simulink model "v2021_10_27_modello_calcolo_trim_1_semplificato"  (R2020b)
settings: Solver=ode4  StartTime=0.0  StopTime=0.01  FixedStep=0.01  RelTol=1e-3
values from neighbouring files (symbols this model uses):
  alphavec_rad = deg2rad(alphavec)    [v2021_10_27_calcoloAerodinamica.m]
  b = 2.62    [v2021_10_27_calcoloAerodinamica.m]
  betavec_rad = deg2rad(betavec)    [v2021_10_27_calcoloAerodinamica.m]
  c = .32    (= 0.32)    [v2021_10_27_calcoloAerodinamica.m]
  cbar = .32    (= 0.32)    [v2021_10_27_calcoloAerodinamica.m]
  CD0 = 0.024    [v2021_10_27_calcoloAerodinamica.m]
  Clp = -0.5058    [v2021_10_27_calcoloAerodinamica.m]
  CLq = 19.166    [v2021_10_27_calcoloAerodinamica.m]
  Clr = 0.1459    [v2021_10_27_calcoloAerodinamica.m]
  Cmq = -81.796    [v2021_10_27_calcoloAerodinamica.m]
  Cnp = 0.007507    [v2021_10_27_calcoloAerodinamica.m]
  Cnr = -1.2593    [v2021_10_27_calcoloAerodinamica.m]
  CYp = 0.050728    [v2021_10_27_calcoloAerodinamica.m]
  CYr = 0.358925    [v2021_10_27_calcoloAerodinamica.m]
  deltaAtrim = 0    [v2021_10_27_avvioSITL.m]
  deltaEtrim = 0    [v2021_10_27_avvioSITL.m]
  deltaRtrim = 0    [v2021_10_27_avvioSITL.m]
  deltaTtrim = 0.1    [v2021_10_27_avvioSITL.m]
  Dprop = 2*Rprop    (= 0.5334)    [v2021_10_27_calcoloAerodinamica.m]
  Jeng = 0    [v2021_10_27_calcoloAerodinamica.m]
  Jprop = mprop*(Dprop^2)/12    (= 0.00422031414)    [v2021_10_27_calcoloAerodinamica.m]
  matricepolinomi = [0.0816560564319 0.0869820125665 0.0279748858868 -4.51852057237 0.0146653626785 -0.925775006168 8.18052218957e-06 -1.47322908992e-05 7.59644694438e-06 0.00246695371279 9.02269223066e-06 0.000559334242525 ... (126 elements, 6x21)]    [coefficienti_curve_renard.mat]
  q = stato(11)    [measure_F1B.m]
  r = stato(12)    [measure_F1B.m]
  rACtG = rACtP-rGP    [v2021_10_27_calcoloAerodinamica.m]
  rACwG = rACwP-rGP    [v2021_10_27_calcoloAerodinamica.m]
  rAHRSG = rAHRSP-rGP    [v2021_10_27_calcoloAerodinamica.m]
  rho = 1.21330    (= 1.2133)    [v2021_10_27_calcoloAerodinamica.m]
  rLEG = rLEP-rGP    [v2021_10_27_calcoloAerodinamica.m]
  rmglG = rmglP-rGP    [v2021_10_27_calcoloAerodinamica.m]
  rmgrG = rmgrP-rGP    [v2021_10_27_calcoloAerodinamica.m]
  rngG = rngP-rGP    [v2021_10_27_calcoloAerodinamica.m]
  rNPG = rNPP-rGP    [v2021_10_27_calcoloAerodinamica.m]
  rPG = -rGP    [v2021_10_27_calcoloAerodinamica.m]
  Rprop = 0.2667    [v2021_10_27_calcoloAerodinamica.m]
  S = b*cbar    (= 0.8384)    [v2021_10_27_calcoloAerodinamica.m]
  W = m*g    [v2021_10_27_calcoloAerodinamica.m]
  Zeng = rPG(3)    [v2021_10_27_calcoloAerodinamica.m]
undefined symbols (not defined in the file or in its folder): CldA, CLdE, CldR, CmdE, CndA, CndR, CYdA, CYdR, F, J_vec, MIL
libraries: aerolibwind2 x3, shared6dof x1, aerolibasang x1, simulink x1
(part 1 of 2)
settings Model: Creator=Giorgio  LastModifiedBy=39334
settings DataIOCC: ReturnWorkspaceOutputs=off
settings OptimizationCC: BlockReduction=off  OptimizeBlockIOStorage=off  BufferReuse=off  GlobalBufferReuse=off  ExpressionFolding=off  LocalBlockOutputs=off  OptimizeDataStoreBuffers=off  BusAssignmentInplaceUpdate=off
settings DebuggingCC: InitInArrayFormatMsg=none  ArithmeticOperatorsInVariantConditions=warning
settings SFSimCC: CustomCodeUndefinedFunction=UseInterfaceOnly

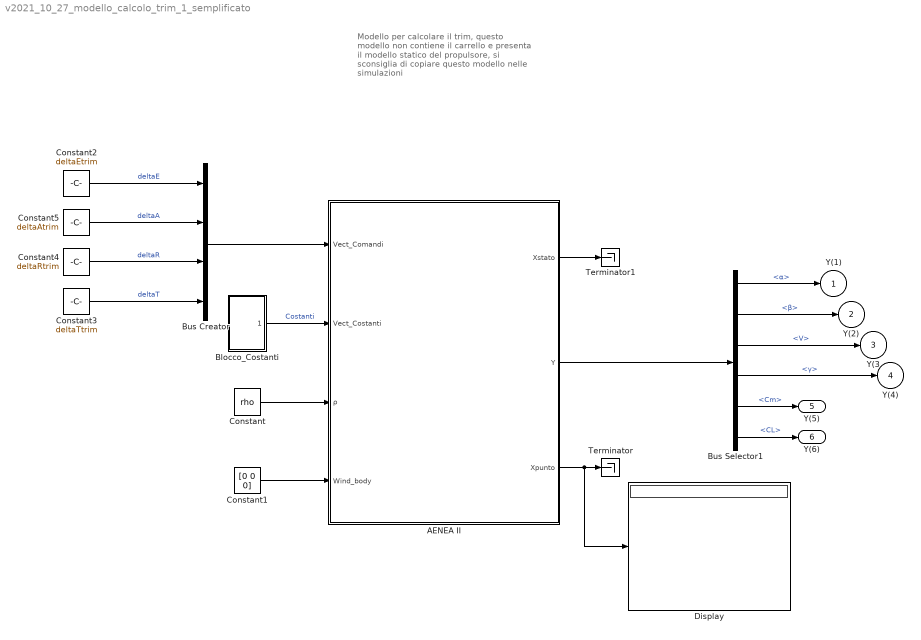
== system v2021_10_27_modello_calcolo_trim_1_semplificato ==
  note: Modello per calcolare il trim, questo modello non contiene il carrello e presenta il modello statico del propulsore, si sconsiglia di copiare questo modello nelle simulazioni
  "AENEA II " : Subsystem
  Blocco_Costanti : Subsystem
  Bus Creator : BusCreator  Inputs=4
  Bus Selector1 : BusSelector  OutputSignals=Vbpolare.α,Vbpolare.β,Vbpolare.V,γ,Cm,CL
  Constant : Constant  Value=rho
  Constant1 : Constant  Value=[0 0 0]
  Constant2 : Constant  Value=deltaEtrim
  Constant3 : Constant  Value=deltaTtrim
  Constant4 : Constant  Value=deltaRtrim
  Constant5 : Constant  Value=deltaAtrim
  Display : Display
  Terminator : Terminator
  Terminator1 : Terminator
  Y(1) : Outport  VectorParamsAs1DForOutWhenUnconnected=off
  Y(2) : Outport  Port=2  VectorParamsAs1DForOutWhenUnconnected=off
  Y(3 : Outport  Port=3  VectorParamsAs1DForOutWhenUnconnected=off
  Y(4) : Outport  Port=4  VectorParamsAs1DForOutWhenUnconnected=off
  Y(5) : Outport  Port=5  VectorParamsAs1DForOutWhenUnconnected=off
  Y(6) : Outport  Port=6  VectorParamsAs1DForOutWhenUnconnected=off
  wires:
  Blocco_Costanti/1(Vect_Costanti) -> "AENEA II "/2(Vect_Costanti)  "Costanti"
  Constant/1 -> "AENEA II "/3(ρ)
  Bus Creator/1 -> "AENEA II "/1(Vect_Comandi)
  Constant5/1 -> Bus Creator/2  "deltaA"
  Constant4/1 -> Bus Creator/3  "deltaR"
  Constant3/1 -> Bus Creator/4  "deltaT"
  Constant2/1 -> Bus Creator/1  "deltaE"
  "AENEA II "/2(Y) -> Bus Selector1/1
  Bus Selector1/1 -> Y(1)/1  "<α>"
  Bus Selector1/2 -> Y(2)/1  "<β>"
  Bus Selector1/3 -> Y(3/1  "<V>"
  Bus Selector1/4 -> Y(4)/1  "<γ>"
  "AENEA II "/1(Xstato) -> Terminator1/1
  Constant1/1 -> "AENEA II "/4(Wind_body)
  "AENEA II "/3(Xpunto) -> Display/1, Terminator/1
  Bus Selector1/5 -> Y(5)/1  "<Cm>"
  Bus Selector1/6 -> Y(6)/1  "<CL>"

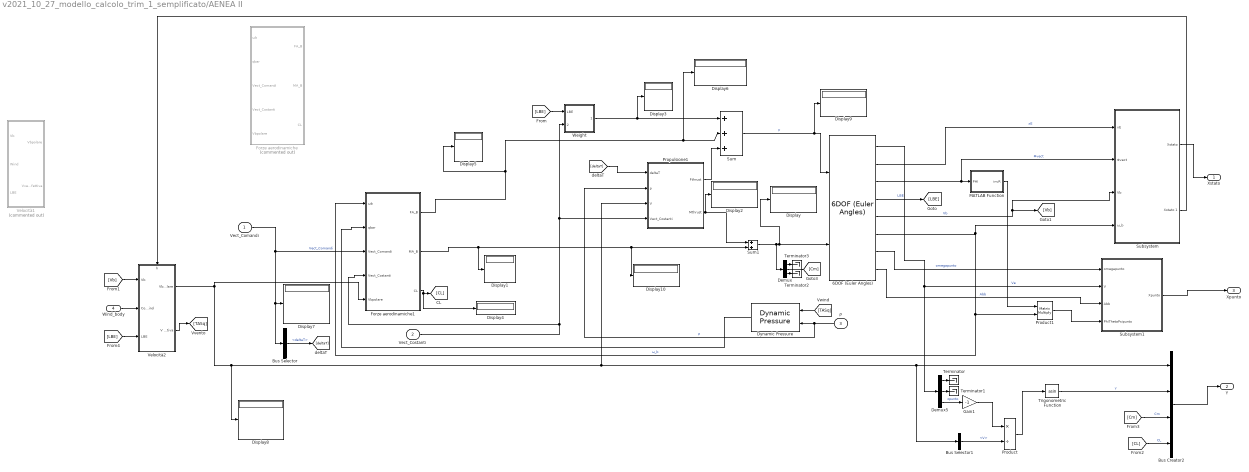
== system v2021_10_27_modello_calcolo_trim_1_semplificato/AENEA II  ==
  Vect_Comandi : Inport
  Vect_Costanti : Inport  Port=2
  ρ : Inport  Port=3
  Wind_body : Inport  Port=4
  6DOF (Euler Angles) : shared6dof/6DOF (Euler Angles)  units=Metric (MKS)  mtype=Fixed  rep=Euler Angles  xme_0=State0.Pos0  Vm_0=State0.Vb0  eul_0=State0.PHI0  pm_0=State0.Omega0  mass_0=m  mass_e=0.5  mass_f=2.0  inertia=I  inertia_e=eye(3)  inertia_f=2*eye(3)  k_quat=1.0  vre_flag=on  abi_flag=off  aMode=aMode  xme_statename=''  Vm_statename=''  eul_statename=''  quat_statename=''  pm_statename=''  mass_statename=''
      settings: SourceProductBaseCode=AE,PW,MT,UV,VE,VP
  Bus Creator2 : BusCreator  Inputs=4
  Bus Selector : BusSelector  OutputSignals=deltaT
  Bus Selector1 : BusSelector  OutputSignals=V
  Demux : Demux  Outputs=3
  Demux5 : Demux  Outputs=3
  Display{,1..10} (11 alike) : Display
  Dynamic Pressure : aerolibasang/Dynamic Pressure
  Forze aerodinamiche : Subsystem  Commented=on
  Forze aerodinamiche1 : Subsystem
  Gain1 : Gain  Gain=-1
  MATLAB Function : MATLAB Function  TreatAsAtomicUnit=on
  Product : Product  Inputs=*/
  Product1 : Product  Multiplication=Matrix(*)
  Propulsione1 : Subsystem
  Subsystem : Subsystem
  Subsystem1 : Subsystem
  Sum : Sum  Inputs=+++
  Sum1 : Sum  Inputs=2
  Terminator{,1..3} (4 alike) : Terminator
  Trigonometric Function : Trigonometry  Operator=asin
  Velocità1 : Subsystem  Commented=on
  Velocità2 : Subsystem
      settings: PortSchema="{\"entries\":[{\"content\":{\"sides\":[{\"content\":{\"connectorIds\":[\"In1\",\"In2\",\"In3\"]},\"type\":\"ConnectorPlacement.EquallySpacedRectSide\",\"uuid\":\"0746aba7-5653-4c82-81e3-16f181e227c2\"},{\"content\":{\"connectorIds\":[\"Out1\",\"Out2\"],\"side\":\"RIGHT\"},\"type\":\"ConnectorPlacement.EquallySpacedRectSide\",\"uuid\":\"8b0f41a9-047a-45e0-b4b5-945564827102\"},{\"content\":{\"connectorIds\":[\"In4\"],\"side\":\"TOP\"},\"type\":\"ConnectorPlacement.EquallySpacedRectSide\",\"uuid\":\"9604396d-4b59-4e8f-8d6f-73032a1dccac\"},{\"content\":{\"connectorIds\":[],\"side\":\"HIDDEN\"},\"type\":\"ConnectorPlacement.EquallySpacedRectSide\",\"uuid\":\"dd1fbc60-e45e-4bfb-a7ae-11fe3343e682\"}]},\"type\":\"ConnectorPlacement.EquallySpacedConnector\",\"uuid\":\"54d3b117-caea-4758-beb0-4ac3e6481041\"}],\"packageUris\":[\"http://schema.mathworks.com/mf0/Connector/R2020b\"],\"version\":\"1.0\"}"
  Weight : Subsystem
  Xstato : Outport  VectorParamsAs1DForOutWhenUnconnected=off
  Y : Outport  Port=2  VectorParamsAs1DForOutWhenUnconnected=off
  Xpunto : Outport  Port=3  VectorParamsAs1DForOutWhenUnconnected=off
  wires:
  Sum/1 -> Display9/1, 6DOF (Euler Angles)/1  "F"
  6DOF (Euler Angles)/5 -> Subsystem/3(Vb), [Vb]  "Vb"
  6DOF (Euler Angles)/6 -> Forze aerodinamiche1/1(ωb), Product1/2, Subsystem/4(ω_b)  "ω_b"
  6DOF (Euler Angles)/4 -> [LBE]  "LBE"
  Forze aerodinamiche1/1(FA_B) -> Sum/2, Display6/1, Display5/1
  Forze aerodinamiche1/2(MA_B) -> Display10/1, Sum1/2, Display1/1
  6DOF (Euler Angles)/1 -> Demux5/1, Subsystem1/2(V)  "Ve"
  Dynamic Pressure/1 -> Forze aerodinamiche1/2(qbar)
  Sum1/1 -> Display/1, 6DOF (Euler Angles)/2, Demux/1
  Weight/1("Forzapeso ") -> Display3/1, Sum/1
  [LBE] -> Weight/1(LBE)
  Vect_Comandi/1 -> Bus Selector/1, Display7/1, Forze aerodinamiche1/3(Vect_Comandi)  "Vect_Comandi"
  Bus Selector/1 -> [deltaT]  "<deltaT>"
  Bus Creator2/1 -> Y/1
  Gain1/1 -> Product/1
  Product/1 -> Trigonometric Function/1
  Trigonometric Function/1 -> Bus Creator2/2  "γ"
  ρ/1 -> Propulsione1/2(ρ), Dynamic Pressure/2  "ρ"
  Velocità2/1(Vbpolare) -> Forze aerodinamiche1/5("Vbpolare "), Display8/1, Propulsione1/3(V), Bus Selector1/1, Bus Creator2/1
  [Vb] -> Velocità2/1(Vb)
  6DOF (Euler Angles)/3 -> Subsystem/2(Φvect), MATLAB Function/1(PHI)  "Φvect"
  Bus Selector1/1 -> Product/2  "<V>"
  Wind_body/1 -> Velocità2/2(Constant Wind)
  Forze aerodinamiche1/3(CL) -> Display4/1, [CL]
  [Cm] -> Bus Creator2/3  "Cm"
  [CL] -> Bus Creator2/4  "CL"
  6DOF (Euler Angles)/2 -> Subsystem/1(xE)  "xE"
  Demux5/2 -> Terminator1/1
  Demux5/1 -> Terminator/1
  Demux5/3 -> Gain1/1  "zpunto"
  6DOF (Euler Angles)/7 -> Subsystem1/1(omegapunto)  "omegapunto"
  6DOF (Euler Angles)/8 -> Subsystem1/3(Abb)  "Abb"
  Subsystem1/1(Xpunto) -> Xpunto/1
  Product1/1 -> Subsystem1/4("PhiThetaPsipunto ")
  MATLAB Function/1(invR) -> Product1/1
  [deltaT] -> Propulsione1/1("deltaT ")
  Vect_Costanti/1 -> Forze aerodinamiche1/4(Vect_Costanti), Propulsione1/4(Vect_Costanti), Weight/2(Vect_Costanti)
  Propulsione1/2(Mthrust) -> Sum1/1, Display2/1
  Propulsione1/1("Fthrust ") -> Sum/3
  Demux/2 -> [Cm]
  Demux/3 -> Terminator2/1
  Demux/1 -> Terminator3/1
  Velocità2/2("V effettiva ") -> [TASq]
  [TASq] -> Dynamic Pressure/1
  [LBE] -> Velocità2/3(LBE)
  Subsystem/1("Xstato ") -> Xstato/1
  Subsystem/2(Xstato 1) -> Velocità2/4(h)

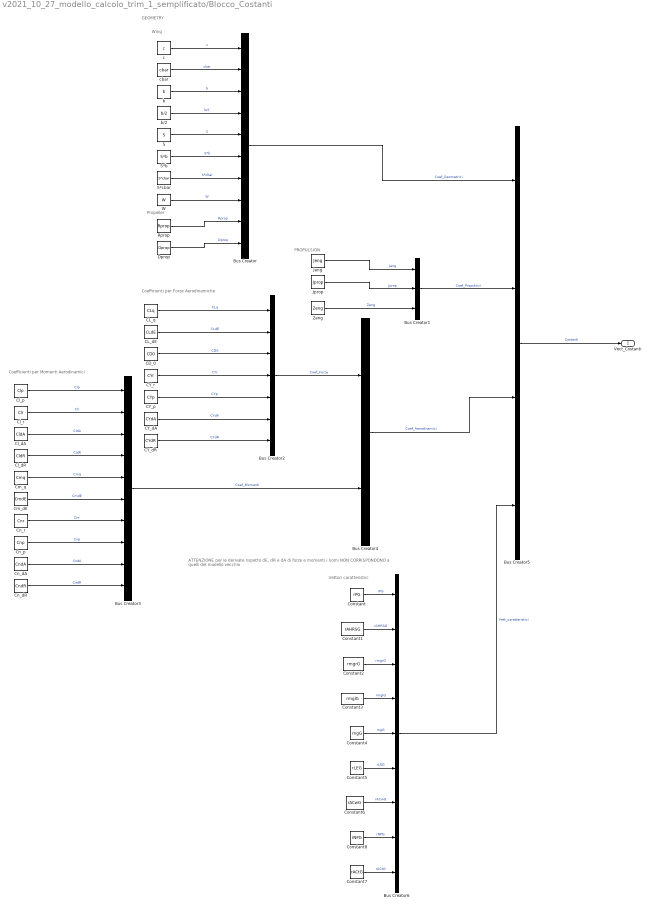
== system v2021_10_27_modello_calcolo_trim_1_semplificato/Blocco_Costanti ==
  note: Vettori caratteristici
  note: ATTENZIONE per le derivate rispetto dE, dR e dA di forze e momenti i nomi NON CORRISPONDONO a quelli del modello vecchio
  note: Coefficienti per Forze Aerodinamiche
  note: Coefficienti per Momenti Aerodinamici
  note: Wing
  note: Propeller
  note: PROPULSION
  note: GEOMETRY
  Bus Creator : BusCreator  Inputs=10
  Bus Creator1 : BusCreator  Inputs=3
  Bus Creator2 : BusCreator  Inputs=7
  Bus Creator3 : BusCreator  Inputs=10
  Bus Creator4 : BusCreator  Inputs=2
  Bus Creator5 : BusCreator  Inputs=4
  Bus Creator6 : BusCreator  Inputs=9
  CD_0 : Constant  Value=CD0
  "CL_dE " : Constant  Value=CLdE
  "CL_q " : Constant  Value=CLq
  CY_dA : Constant  Value=CYdA
  CY_dR : Constant  Value=CYdR
  "CY_p " : Constant  Value=CYp
  CY_r : Constant  Value=CYr
  Cl_dA : Constant  Value=CldA
  Cl_dR : Constant  Value=CldR
  "Cl_p " : Constant  Value=Clp
  "Cl_r " : Constant  Value=Clr
  "Cm_dE " : Constant  Value=CmdE
  "Cm_q " : Constant  Value=Cmq
  Cn_dA : Constant  Value=CndA
  "Cn_dR " : Constant  Value=CndR
  "Cn_p " : Constant  Value=Cnp
  "Cn_r " : Constant  Value=Cnr
  Constant : Constant  Value=rPG
  Constant1 : Constant  Value=rAHRSG
  Constant2 : Constant  Value=rmgrG
  Constant3 : Constant  Value=rmglG
  Constant4 : Constant  Value=rngG
  Constant5 : Constant  Value=rLEG
  Constant6 : Constant  Value=rACwG
  Constant7 : Constant  Value=rACtG
  Constant8 : Constant  Value=rNPG
  Dprop : Constant  Value=Dprop
  Jeng : Constant  Value=Jeng
  Jprop : Constant  Value=Jprop
  Rprop : Constant  Value=Rprop
  S : Constant  Value=S
  "S*b " : Constant  Value=S*b
  S*cbar : Constant  Value=S*cbar
  W : Constant  Value=W
  Zeng : Constant  Value=Zeng
  b : Constant  Value=b
  b/2 : Constant  Value=b/2
  c : Constant  Value=c
  "cbar " : Constant  Value=cbar
  Vect_Costanti : Outport  VectorParamsAs1DForOutWhenUnconnected=off
  wires:
  "CY_p "/1 -> Bus Creator2/5  "CYp"
  Cl_dR/1 -> Bus Creator3/4  "CldR"
  "Cn_dR "/1 -> Bus Creator3/10  "CndR"
  "CL_q "/1 -> Bus Creator2/1  "CLq"
  "Cn_p "/1 -> Bus Creator3/8  "Cnp"
  Bus Creator1/1 -> Bus Creator5/2  "Coef_Propulsivi"
  CD_0/1 -> Bus Creator2/3  "CD0"
  Bus Creator4/1 -> Bus Creator5/3  "Coef_Aerodinamici"
  "Cm_dE "/1 -> Bus Creator3/6  "CmdE"
  "Cn_r "/1 -> Bus Creator3/7  "Cnr"
  "Cl_r "/1 -> Bus Creator3/2  "Clr"
  "Cm_q "/1 -> Bus Creator3/5  "Cmq"
  CY_dR/1 -> Bus Creator2/7  "CYdR"
  Cl_dA/1 -> Bus Creator3/3  "CldA"
  CY_dA/1 -> Bus Creator2/6  "CYdA"
  "CL_dE "/1 -> Bus Creator2/2  "CLdE"
  Dprop/1 -> Bus Creator/10  "Dprop"
  Cn_dA/1 -> Bus Creator3/9  "CndA"
  Bus Creator5/1 -> Vect_Costanti/1  "Costanti"
  Bus Creator/1 -> Bus Creator5/1  "Coef_Geometrici"
  Jeng/1 -> Bus Creator1/1  "Jeng"
  c/1 -> Bus Creator/1  "c"
  "S*b "/1 -> Bus Creator/6  "S*b"
  W/1 -> Bus Creator/8  "W"
  Rprop/1 -> Bus Creator/9  "Rprop"
  b/1 -> Bus Creator/3  "b"
  Bus Creator3/1 -> Bus Creator4/2  "Coef_Momenti"
  Bus Creator2/1 -> Bus Creator4/1  "Coef_Forze"
  S*cbar/1 -> Bus Creator/7  "S*cbar"
  Jprop/1 -> Bus Creator1/2  "Jprop"
  b/2/1 -> Bus Creator/4  "b/2"
  "Cl_p "/1 -> Bus Creator3/1  "Clp"
  CY_r/1 -> Bus Creator2/4  "CYr"
  S/1 -> Bus Creator/5  "S"
  "cbar "/1 -> Bus Creator/2  "cbar"
  Zeng/1 -> Bus Creator1/3  "Zeng"
  Constant/1 -> Bus Creator6/1  "rPG"
  Bus Creator6/1 -> Bus Creator5/4  "Vett_caratteristici"
  Constant3/1 -> Bus Creator6/4  "rmglG"
  Constant8/1 -> Bus Creator6/8  "rNPG"
  Constant6/1 -> Bus Creator6/7  "rACwG"
  Constant5/1 -> Bus Creator6/6  "rLEG"
  Constant4/1 -> Bus Creator6/5  "rngG"
  Constant7/1 -> Bus Creator6/9  "rACtG"
  Constant2/1 -> Bus Creator6/3  "rmgrG"
  Constant1/1 -> Bus Creator6/2  "rAHRSG"

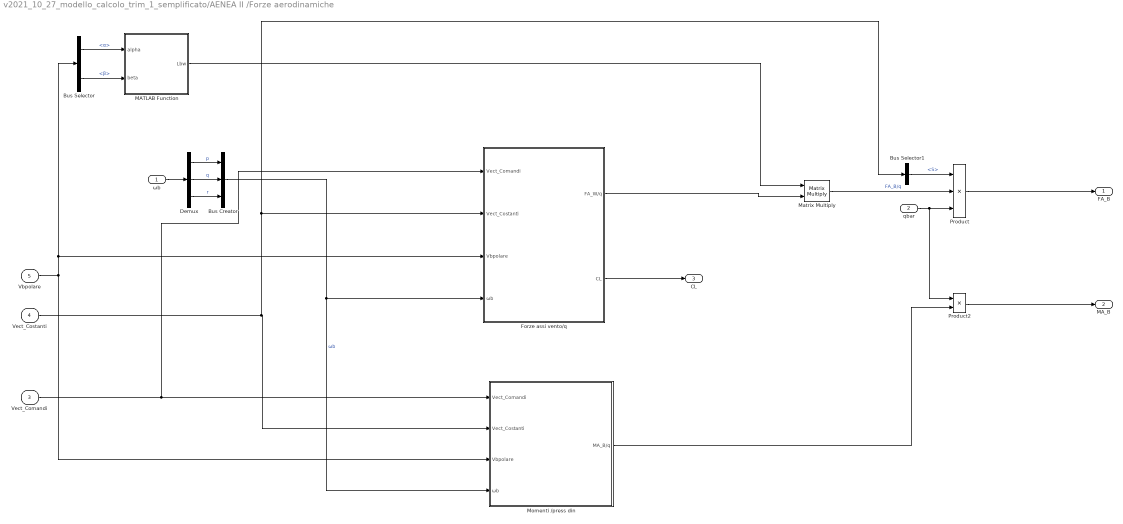
== system v2021_10_27_modello_calcolo_trim_1_semplificato/AENEA II /Forze aerodinamiche ==
  ωb : Inport
  qbar : Inport  Port=2
  Vect_Comandi : Inport  Port=3
  Vect_Costanti : Inport  Port=4
  "Vbpolare " : Inport  Port=5
  Bus Creator : BusCreator  Inputs=3
  Bus Selector : BusSelector  OutputSignals=α,β
  Bus Selector1 : BusSelector  OutputSignals=Coef_Geometrici.S
  Demux : Demux  Outputs=3
  Forze assi vento/q : Subsystem
  MATLAB Function : MATLAB Function  TreatAsAtomicUnit=on
  Matrix Multiply : Product  Multiplication=Matrix(*)
  Momenti /press din : Subsystem
  Product : Product  Inputs=3
  Product2 : Product
  FA_B : Outport  VectorParamsAs1DForOutWhenUnconnected=off
  MA_B : Outport  Port=2  VectorParamsAs1DForOutWhenUnconnected=off
  CL : Outport  Port=3  VectorParamsAs1DForOutWhenUnconnected=off
  wires:
  Product2/1 -> MA_B/1
  Product/1 -> FA_B/1
  qbar/1 -> Product/3, Product2/1
  ωb/1 -> Demux/1
  Demux/1 -> Bus Creator/1  "p"
  Demux/2 -> Bus Creator/2  "q"
  Demux/3 -> Bus Creator/3  "r"
  Bus Selector/1 -> MATLAB Function/1(alpha)  "<α>"
  Bus Selector/2 -> MATLAB Function/2(beta)  "<β>"
  MATLAB Function/1(Lbw) -> Matrix Multiply/1
  Matrix Multiply/1 -> Product/2  "FA_B/q"
  Momenti /press din/1(MA_B/q) -> Product2/2
  Forze assi vento/q/1(FA_W/q) -> Matrix Multiply/2
  Vect_Comandi/1 -> Forze assi vento/q/1(Vect_Comandi), Momenti /press din/1(Vect_Comandi)
  "Vbpolare "/1 -> Bus Selector/1, Forze assi vento/q/3("Vbpolare "), Momenti /press din/3("Vbpolare ")
  Bus Creator/1 -> Momenti /press din/4(ωb), Forze assi vento/q/4(ωb)  "ωb"
  Vect_Costanti/1 -> Bus Selector1/1, Forze assi vento/q/2(Vect_Costanti), Momenti /press din/2(Vect_Costanti)
  Bus Selector1/1 -> Product/1  "<S>"
  Forze assi vento/q/2(CL) -> CL/1

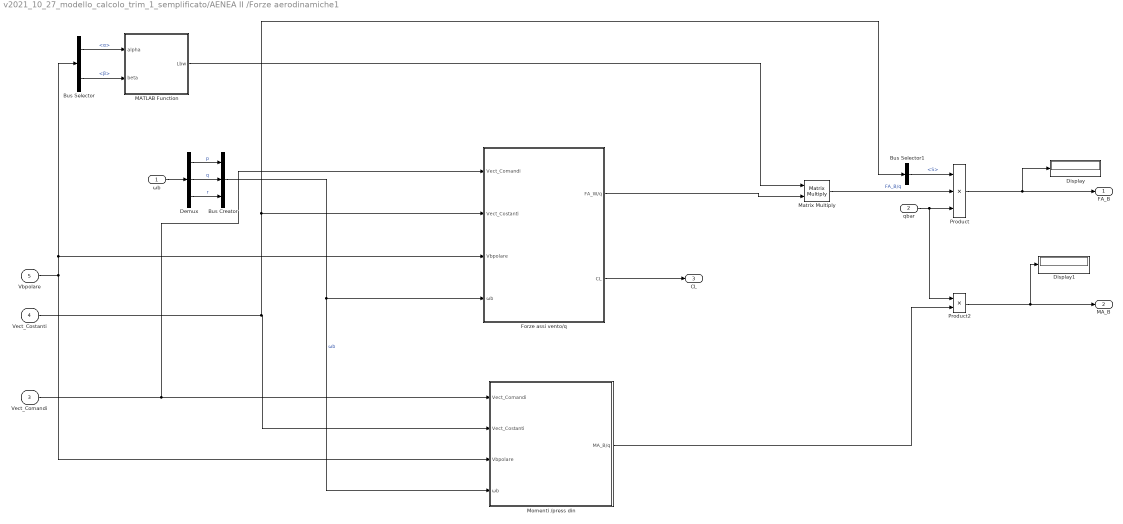
== system v2021_10_27_modello_calcolo_trim_1_semplificato/AENEA II /Forze aerodinamiche1 ==
  ωb : Inport
  qbar : Inport  Port=2
  Vect_Comandi : Inport  Port=3
  Vect_Costanti : Inport  Port=4
  "Vbpolare " : Inport  Port=5
  Bus Creator : BusCreator  Inputs=3
  Bus Selector : BusSelector  OutputSignals=α,β
  Bus Selector1 : BusSelector  OutputSignals=Coef_Geometrici.S
  Demux : Demux  Outputs=3
  Display : Display
  Display1 : Display
  Forze assi vento/q : Subsystem
  MATLAB Function : MATLAB Function  TreatAsAtomicUnit=on
  Matrix Multiply : Product  Multiplication=Matrix(*)
  Momenti /press din : Subsystem
  Product : Product  Inputs=3
  Product2 : Product
  FA_B : Outport  VectorParamsAs1DForOutWhenUnconnected=off
  MA_B : Outport  Port=2  VectorParamsAs1DForOutWhenUnconnected=off
  CL : Outport  Port=3  VectorParamsAs1DForOutWhenUnconnected=off
  wires:
  Product2/1 -> Display1/1, MA_B/1
  Product/1 -> Display/1, FA_B/1
  qbar/1 -> Product/3, Product2/1
  ωb/1 -> Demux/1
  Demux/1 -> Bus Creator/1  "p"
  Demux/2 -> Bus Creator/2  "q"
  Demux/3 -> Bus Creator/3  "r"
  Bus Selector/1 -> MATLAB Function/1(alpha)  "<α>"
  Bus Selector/2 -> MATLAB Function/2(beta)  "<β>"
  MATLAB Function/1(Lbw) -> Matrix Multiply/1
  Matrix Multiply/1 -> Product/2  "FA_B/q"
  Momenti /press din/1(MA_B/q) -> Product2/2
  Forze assi vento/q/1(FA_W/q) -> Matrix Multiply/2
  Vect_Comandi/1 -> Forze assi vento/q/1(Vect_Comandi), Momenti /press din/1(Vect_Comandi)
  "Vbpolare "/1 -> Bus Selector/1, Forze assi vento/q/3("Vbpolare "), Momenti /press din/3("Vbpolare ")
  Bus Creator/1 -> Momenti /press din/4(ωb), Forze assi vento/q/4(ωb)  "ωb"
  Vect_Costanti/1 -> Bus Selector1/1, Forze assi vento/q/2(Vect_Costanti), Momenti /press din/2(Vect_Costanti)
  Bus Selector1/1 -> Product/1  "<S>"
  Forze assi vento/q/2(CL) -> CL/1

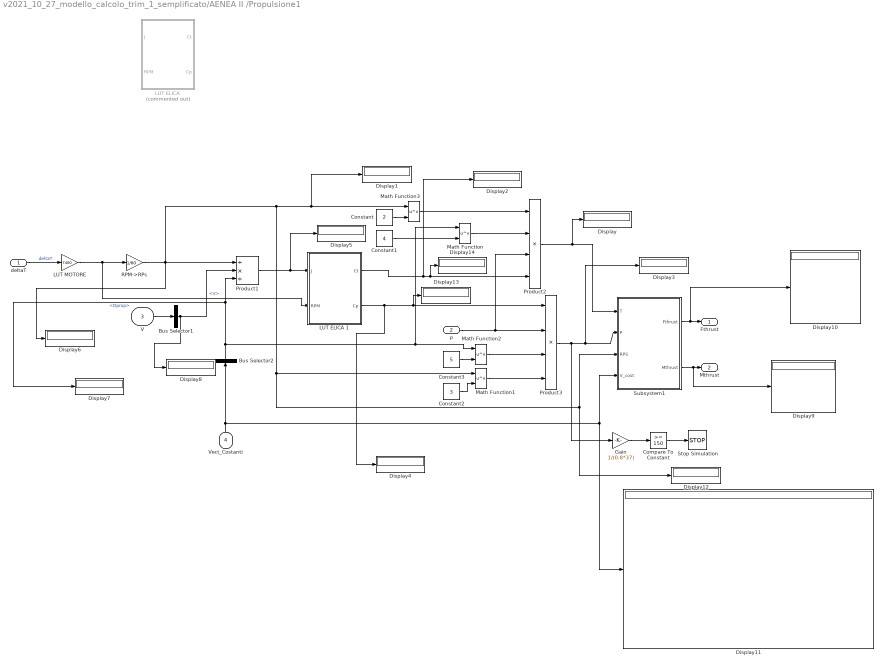
== system v2021_10_27_modello_calcolo_trim_1_semplificato/AENEA II /Propulsione1 ==
  "deltaT " : Inport
  ρ : Inport  Port=2
  V : Inport  Port=3
  Vect_Costanti : Inport  Port=4
  Bus Selector1 : BusSelector  OutputSignals=V
  Bus Selector2 : BusSelector  OutputSignals=Coef_Geometrici.Dprop
  Compare To Constant : simulink/Logic and Bit Operations/Compare To Constant  relop=>=  const=150  OutDataTypeStr=boolean
  Constant : Constant  Value=2
  Constant1 : Constant  Value=4
  Constant2 : Constant  Value=3
  Constant3 : Constant  Value=5
  Display{,1..14} (15 alike) : Display
  Gain : Gain  Gain=1/(0.8*37)
  "LUT ELICA " : Subsystem  Commented=on
  LUT ELICA 1 : Subsystem
  LUT MOTORE : Gain  Gain=7400
  Math Function{,1..3} (4 alike) : Math  Operator=pow  SignedPower=on  SaturateOnIntegerOverflow=on
  Product1 : Product  Inputs=/*/
  Product2 : Product  Inputs=****
  Product3 : Product  Inputs=****
  RPM->RPs : Gain  Gain=1/60
  Stop Simulation : Stop
  Subsystem1 : Subsystem
  "Fthrust " : Outport  VectorParamsAs1DForOutWhenUnconnected=off
  Mthrust : Outport  Port=2  VectorParamsAs1DForOutWhenUnconnected=off
  wires:
  Vect_Costanti/1 -> Display11/1, Subsystem1/4(V_cost), Bus Selector2/1
  "deltaT "/1 -> LUT MOTORE/1  "deltaT"
  LUT MOTORE/1 -> LUT ELICA 1/2(RPM), RPM->RPs/1
  V/1 -> Bus Selector1/1
  Bus Selector1/1 -> Display8/1, Product1/2  "<V>"
  RPM->RPs/1 -> Display6/1, Product1/1, Display12/1, Subsystem1/3(RPS), Math Function1/1, Display1/1, Math Function3/1
  Bus Selector2/1 -> Display7/1, Product1/3, Math Function2/1, Math Function/1  "<Dprop>"
  Product1/1 -> LUT ELICA 1/1(J), Display5/1
  ρ/1 -> Product2/3, Product3/2
  LUT ELICA 1/2(Cp) -> Display4/1, Display13/1, Product3/1
  LUT ELICA 1/1(Ct) -> Display2/1, Display14/1, Product2/4
  Math Function3/1 -> Product2/1
  Math Function/1 -> Product2/2
  Constant/1 -> Math Function3/2
  Constant1/1 -> Math Function/2
  Math Function2/1 -> Product3/3
  Constant3/1 -> Math Function2/2
  Constant2/1 -> Math Function1/2
  Math Function1/1 -> Product3/4
  Product2/1 -> Display/1, Subsystem1/1(T)
  Subsystem1/1(Fthrust) -> Display10/1, "Fthrust "/1
  Subsystem1/2("Mthrust ") -> Display9/1, Mthrust/1
  Product3/1 -> Gain/1, Display3/1, Subsystem1/2(P)
  Gain/1 -> Compare To Constant/1
  Compare To Constant/1 -> Stop Simulation/1

== system v2021_10_27_modello_calcolo_trim_1_semplificato/AENEA II /Subsystem ==
  xE : Inport
  Φvect : Inport  Port=2
  Vb : Inport  Port=3
  ω_b : Inport  Port=4
  Bus Creator1 : BusCreator  Inputs=4
  Bus Creator{3..4,8..9} (4 alike) : BusCreator  Inputs=3
  Demux{1..2,6..7} (4 alike) : Demux  Outputs=3
  "Xstato " : Outport  VectorParamsAs1DForOutWhenUnconnected=off
  Xstato 1 : Outport  Port=2  VectorParamsAs1DForOutWhenUnconnected=off
  wires:
  Demux2/3 -> Bus Creator4/3  "r"
  Bus Creator4/1 -> Bus Creator1/3  "ωvect"
  Φvect/1 -> Demux6/1
  Vb/1 -> Demux7/1
  Bus Creator8/1 -> Bus Creator1/2  "PhiThetaPsi"
  Demux1/3 -> Xstato 1/1, Bus Creator3/3  "h"
  Demux2/2 -> Bus Creator4/2  "q"
  Demux2/1 -> Bus Creator4/1  "p"
  Bus Creator3/1 -> Bus Creator1/4  "xyz"
  ω_b/1 -> Demux2/1
  Demux6/3 -> Bus Creator8/3  "Psi"
  Demux6/1 -> Bus Creator8/1  "Phi"
  Demux1/1 -> Bus Creator3/1  "x"
  Demux7/1 -> Bus Creator9/1  "u"
  Demux7/3 -> Bus Creator9/3  "w"
  Bus Creator9/1 -> Bus Creator1/1  "uvw"
  Demux1/2 -> Bus Creator3/2  "y"
  Demux7/2 -> Bus Creator9/2  "v"
  Demux6/2 -> Bus Creator8/2  "Theta"
  Bus Creator1/1 -> "Xstato "/1  "Xstato"
  xE/1 -> Demux1/1

== system v2021_10_27_modello_calcolo_trim_1_semplificato/AENEA II /Subsystem1 ==
  omegapunto : Inport
  V : Inport  Port=2
  Abb : Inport  Port=3
  "PhiThetaPsipunto " : Inport  Port=4
  Bus Creator{5,7,10..11} (4 alike) : BusCreator  Inputs=3
  Bus Creator6 : BusCreator  Inputs=4
  Demux{3..4,8..9} (4 alike) : Demux  Outputs=3
  Xpunto : Outport  VectorParamsAs1DForOutWhenUnconnected=off
  wires:
  Demux4/3 -> Bus Creator7/3  "wpunto"
  Demux3/1 -> Bus Creator5/1  "ppunto"
  Demux4/2 -> Bus Creator7/2  "vpunto"
  Demux8/2 -> Bus Creator10/2  "Thetapunto"
  Bus Creator10/1 -> Bus Creator6/2  "EulerAnglespunto"
  Demux3/2 -> Bus Creator5/2  "qpunto"
  Demux4/1 -> Bus Creator7/1  "upunto"
  V/1 -> Demux9/1
  Demux8/1 -> Bus Creator10/1  "Phipunto"
  Bus Creator11/1 -> Bus Creator6/4  "xyzpunto"
  Demux8/3 -> Bus Creator10/3  "Psipunto"
  Demux3/3 -> Bus Creator5/3  "rpunto"
  Demux9/2 -> Bus Creator11/2  "Yepunto"
  Bus Creator7/1 -> Bus Creator6/1  "Vbpunto"
  Bus Creator5/1 -> Bus Creator6/3  "ωpunto"
  Demux9/1 -> Bus Creator11/1  "Xepunto"
  Demux9/3 -> Bus Creator11/3  "Zepunto"
  "PhiThetaPsipunto "/1 -> Demux8/1
  omegapunto/1 -> Demux3/1
  Abb/1 -> Demux4/1
  Bus Creator6/1 -> Xpunto/1

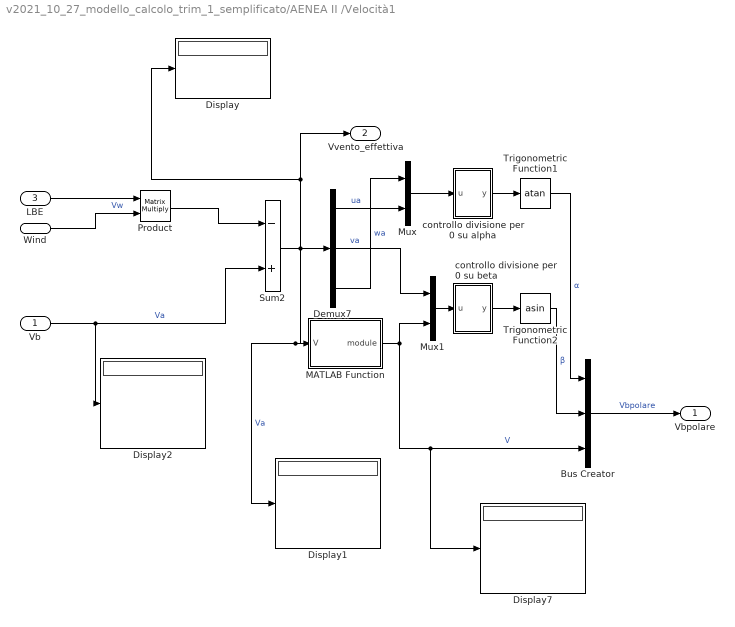
== system v2021_10_27_modello_calcolo_trim_1_semplificato/AENEA II /Velocità1 ==
  Vb : Inport
  Wind : Inport  Port=2
  LBE : Inport  Port=3
  Bus Creator : BusCreator  Inputs=3
  Demux7 : Demux  Outputs=3
  Display{,1..2,7} (4 alike) : Display
  MATLAB Function : MATLAB Function  TreatAsAtomicUnit=on
  Mux : Mux  Inputs=2
  Mux1 : Mux  Inputs=2
  Product : Product  Multiplication=Matrix(*)
  Sum2 : Sum  Inputs=-+
  Trigonometric Function1 : Trigonometry  Operator=atan
  Trigonometric Function2 : Trigonometry  Operator=asin
  controllo divisione per 0 su alpha : MATLAB Function  TreatAsAtomicUnit=on
  controllo divisione per 0 su beta : MATLAB Function  TreatAsAtomicUnit=on
  Vbpolare : Outport  VectorParamsAs1DForOutWhenUnconnected=off
  "Vvento_effettiva " : Outport  Port=2  VectorParamsAs1DForOutWhenUnconnected=off
  wires:
  Bus Creator/1 -> Vbpolare/1  "Vbpolare"
  Trigonometric Function1/1 -> Bus Creator/1  "α"
  MATLAB Function/1(module) -> Mux1/2, Display7/1, Bus Creator/3  "V"
  controllo divisione per 0 su alpha/1(y) -> Trigonometric Function1/1
  controllo divisione per 0 su beta/1(y) -> Trigonometric Function2/1
  Trigonometric Function2/1 -> Bus Creator/2  "β"
  Vb/1 -> Display2/1, Sum2/2  "Va"
  Sum2/1 -> Display/1, "Vvento_effettiva "/1, Demux7/1, Display1/1, MATLAB Function/1(V)  "Va"
  Mux/1 -> controllo divisione per 0 su alpha/1(u)
  Demux7/3 -> Mux/1  "wa"
  Demux7/1 -> Mux/2  "ua"
  Mux1/1 -> controllo divisione per 0 su beta/1(u)
  Demux7/2 -> Mux1/1  "va"
  Wind/1 -> Product/2  "Vw"
  LBE/1 -> Product/1
  Product/1 -> Sum2/1

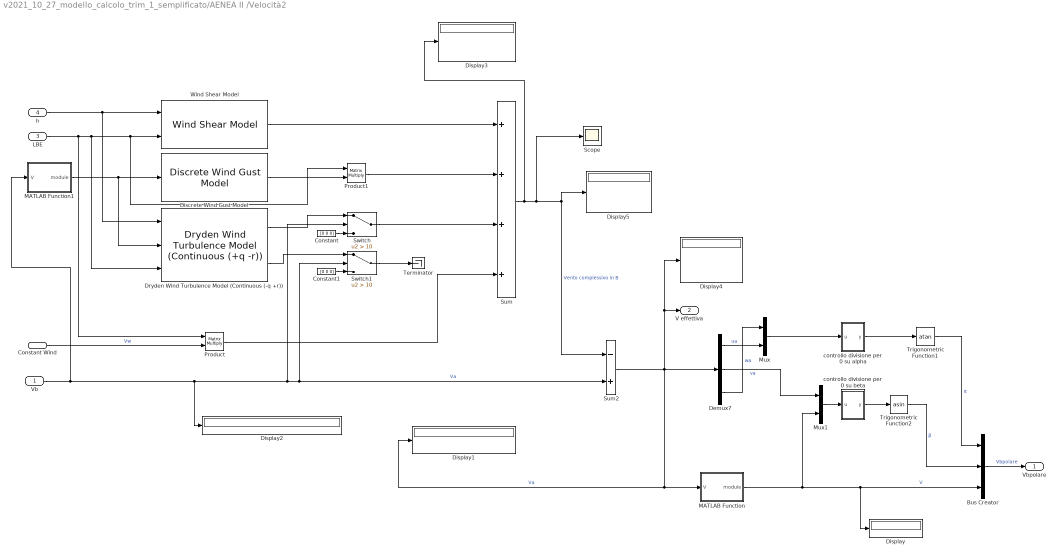
== system v2021_10_27_modello_calcolo_trim_1_semplificato/AENEA II /Velocità2 ==
  Vb : Inport
  Constant Wind : Inport  Port=2
  LBE : Inport  Port=3
  h : Inport  Port=4
  Bus Creator : BusCreator  Inputs=3
  Constant : Constant  Value=[0 0 0]
  Constant1 : Constant  Value=[0 0 0]
  Demux7 : Demux  Outputs=3
  Discrete Wind Gust Model : aerolibwind2/Discrete Wind Gust Model  units=Metric (MKS)  Gx=on  Gy=on  Gz=on  t_0=80  d_m=[120 120 80]  v_m=[0 0 0]
  Display{,1..5} (6 alike) : Display
  Dryden Wind Turbulence Model (Continuous (-q +r)) : aerolibwind2/Dryden Wind Turbulence Model  (Continuous (+q -r))  units=Metric (MKS)  spec=MIL-F-8785C  model=Continuous Dryden (-q +r)  W20=0  Wdeg=180  TurbProb=10^-4  L_high=533.4  Wingspan=2.6  ts=0.01  Seed=[23341 23342 23343 23344]  T_on=on
  MATLAB Function : MATLAB Function  TreatAsAtomicUnit=on
  MATLAB Function1 : MATLAB Function  TreatAsAtomicUnit=on
  Mux : Mux  Inputs=2
  Mux1 : Mux  Inputs=2
  Product : Product  Multiplication=Matrix(*)
  Product1 : Product  Multiplication=Matrix(*)
  Scope : Scope
  Sum : Sum  Inputs=4
  Sum2 : Sum  Inputs=-+
  Switch : Switch  Criteria=u2 > Threshold  Threshold=10
  Switch1 : Switch  Criteria=u2 > Threshold  Threshold=10
  Terminator : Terminator
  Trigonometric Function1 : Trigonometry  Operator=atan
  Trigonometric Function2 : Trigonometry  Operator=asin
  Wind Shear Model : aerolibwind2/Wind Shear Model  units=Metric (MKS)  phase=Category C - Terminal Flight Phase  W_20=0  Wdeg=180
  controllo divisione per 0 su alpha : MATLAB Function  TreatAsAtomicUnit=on
  controllo divisione per 0 su beta : MATLAB Function  TreatAsAtomicUnit=on
  Vbpolare : Outport  VectorParamsAs1DForOutWhenUnconnected=off
  "V effettiva " : Outport  Port=2  VectorParamsAs1DForOutWhenUnconnected=off
  wires:
  Bus Creator/1 -> Vbpolare/1  "Vbpolare"
  Trigonometric Function1/1 -> Bus Creator/1  "α"
  MATLAB Function/1(module) -> Mux1/2, Display/1, Bus Creator/3  "V"
  controllo divisione per 0 su alpha/1(y) -> Trigonometric Function1/1
  controllo divisione per 0 su beta/1(y) -> Trigonometric Function2/1
  Trigonometric Function2/1 -> Bus Creator/2  "β"
  Vb/1 -> Display2/1, Switch/2, Switch1/2, Sum2/2, MATLAB Function1/1(V)  "Va"
  Sum2/1 -> "V effettiva "/1, Display4/1, Demux7/1, Display1/1, MATLAB Function/1(V)  "Va"
  Mux/1 -> controllo divisione per 0 su alpha/1(u)
  Demux7/3 -> Mux/1  "wa"
  Demux7/1 -> Mux/2  "ua"
  Mux1/1 -> controllo divisione per 0 su beta/1(u)
  Demux7/2 -> Mux1/1  "va"
  Constant Wind/1 -> Product/2  "Vw"
  h/1 -> Dryden Wind Turbulence Model (Continuous (-q +r))/1, Wind Shear Model/1
  LBE/1 -> Product/1, Dryden Wind Turbulence Model (Continuous (-q +r))/3, Product1/1, Wind Shear Model/2
  Dryden Wind Turbulence Model (Continuous (-q +r))/1 -> Switch/1
  Constant/1 -> Switch/3
  Dryden Wind Turbulence Model (Continuous (-q +r))/2 -> Switch1/1
  Constant1/1 -> Switch1/3
  Wind Shear Model/1 -> Sum/1
  Discrete Wind Gust Model/1 -> Product1/2
  Product1/1 -> Sum/2
  Switch/1 -> Sum/3
  Switch1/1 -> Terminator/1
  Product/1 -> Sum/4
  Sum/1 -> Display3/1, Scope/1, Display5/1, Sum2/1  "Vento complessivo in B"
  MATLAB Function1/1(module) -> Dryden Wind Turbulence Model (Continuous (-q +r))/2, Discrete Wind Gust Model/1

== system v2021_10_27_modello_calcolo_trim_1_semplificato/AENEA II /Weight ==
  LBE : Inport
  Vect_Costanti : Inport  Port=2
  Bus Selector : BusSelector  OutputSignals=Coef_Geometrici.W
  Display3 : Display
  Product3 : Product  Multiplication=Matrix(*)
  "Forzapeso " : Outport  VectorParamsAs1DForOutWhenUnconnected=off
  wires:
  Product3/1 -> "Forzapeso "/1, Display3/1
  LBE/1 -> Product3/1
  Vect_Costanti/1 -> Bus Selector/1
  Bus Selector/1 -> Product3/2  "<W>"

== system v2021_10_27_modello_calcolo_trim_1_semplificato/AENEA II /Forze aerodinamiche/Forze assi vento//q ==
  Vect_Comandi : Inport
  Vect_Costanti : Inport  Port=2
  "Vbpolare " : Inport  Port=3
  ωb : Inport  Port=4
  Bus Creator : BusCreator  Inputs=3
  Bus Selector : BusSelector  OutputSignals=deltaE
  Bus Selector1 : BusSelector  OutputSignals=p,r,q
  Display : Display
  Gain4 : Gain  Gain=-1
  Gain5 : Gain  Gain=-1
  Scope : Scope
  Subsystem : Subsystem
  Subsystem1 : Subsystem
  Subsystem2 : Subsystem
  FA_W/q : Outport  VectorParamsAs1DForOutWhenUnconnected=off
  CL : Outport  Port=2  VectorParamsAs1DForOutWhenUnconnected=off
  wires:
  Bus Selector/1 -> Subsystem2/2(deltaE)  "<deltaE>"
  Subsystem/1(CD) -> Display/1, Scope/1, Gain4/1
  Subsystem2/1(CL) -> CL/1, Gain5/1
  Vect_Costanti/1 -> Subsystem2/3(Vect_Costanti), Subsystem1/3(Vect_Costanti), Subsystem/1(Vect_Costanti)
  Vect_Comandi/1 -> Subsystem1/4(Vect_Comandi), Bus Selector/1
  "Vbpolare "/1 -> Subsystem1/5("Vbpolare "), Subsystem2/4("Vbpolare "), Subsystem/2("Vbpolare ")
  ωb/1 -> Bus Selector1/1
  Bus Selector1/1 -> Subsystem1/1(p)  "<p>"
  Bus Selector1/3 -> Subsystem2/1(q)  "<q>"
  Bus Selector1/2 -> Subsystem1/2(r)  "<r>"
  Bus Creator/1 -> FA_W/q/1
  Gain5/1 -> Bus Creator/3  "CL"
  Subsystem1/1("CY ") -> Bus Creator/2  "CY"
  Gain4/1 -> Bus Creator/1  "CD"

== system v2021_10_27_modello_calcolo_trim_1_semplificato/AENEA II /Forze aerodinamiche/Momenti //press din ==
  Vect_Comandi : Inport
  Vect_Costanti : Inport  Port=2
  "Vbpolare " : Inport  Port=3
  ωb : Inport  Port=4
  Bus Creator : BusCreator  Inputs=3
  Bus Selector : BusSelector  OutputSignals=Coef_Geometrici.S*b,Coef_Geometrici.S*cbar
  Product : Product
  Product1 : Product
  Product3 : Product
  Subsystem3 : Subsystem
  Subsystem4 : Subsystem
  Subsystem5 : Subsystem
  MA_B/q : Outport  VectorParamsAs1DForOutWhenUnconnected=off
  wires:
  Subsystem5/1(Cn) -> Product3/2
  Subsystem4/1(Cm) -> Product1/2
  Subsystem3/1(Cl) -> Product/2
  Vect_Costanti/1 -> Bus Selector/1, Subsystem3/1(Vect_Costanti), Subsystem5/1(Vect_Costanti), Subsystem4/1(Vect_Costanti)
  Vect_Comandi/1 -> Subsystem4/2(Vect_Comandi), Subsystem3/2(Vect_Comandi), Subsystem5/2(Vect_Comandi)
  "Vbpolare "/1 -> Subsystem5/3("Vbpolare "), Subsystem4/3("Vbpolare "), Subsystem3/3("Vbpolare ")
  ωb/1 -> Subsystem5/4(ωb), Subsystem4/4(ωb), Subsystem3/4(ωb)
  Bus Selector/1 -> Product3/1, Product/1  "<S*b>"
  Bus Selector/2 -> Product1/1  "<S*cbar>"
  Bus Creator/1 -> MA_B/q/1
  Product/1 -> Bus Creator/1  "Cl"
  Product1/1 -> Bus Creator/2  "Cm"
  Product3/1 -> Bus Creator/3  "Cn"

== system v2021_10_27_modello_calcolo_trim_1_semplificato/AENEA II /Forze aerodinamiche1/Forze assi vento//q ==
  Vect_Comandi : Inport
  Vect_Costanti : Inport  Port=2
  "Vbpolare " : Inport  Port=3
  ωb : Inport  Port=4
  Bus Creator : BusCreator  Inputs=3
  Bus Selector : BusSelector  OutputSignals=deltaE
  Bus Selector1 : BusSelector  OutputSignals=p,r,q
  Display : Display
  Gain4 : Gain  Gain=-1
  Gain5 : Gain  Gain=-1
  Scope : Scope
  Subsystem : Subsystem
  Subsystem1 : Subsystem
  Subsystem2 : Subsystem
  FA_W/q : Outport  VectorParamsAs1DForOutWhenUnconnected=off
  CL : Outport  Port=2  VectorParamsAs1DForOutWhenUnconnected=off
  wires:
  Bus Selector/1 -> Subsystem2/2(deltaE)  "<deltaE>"
  Subsystem/1(CD) -> Display/1, Scope/1, Gain4/1
  Subsystem2/1(CL) -> CL/1, Gain5/1
  Vect_Costanti/1 -> Subsystem2/3(Vect_Costanti), Subsystem1/3(Vect_Costanti), Subsystem/1(Vect_Costanti)
  Vect_Comandi/1 -> Subsystem1/4(Vect_Comandi), Bus Selector/1
  "Vbpolare "/1 -> Subsystem1/5("Vbpolare "), Subsystem2/4("Vbpolare "), Subsystem/2("Vbpolare ")
  ωb/1 -> Bus Selector1/1
  Bus Selector1/1 -> Subsystem1/1(p)  "<p>"
  Bus Selector1/3 -> Subsystem2/1(q)  "<q>"
  Bus Selector1/2 -> Subsystem1/2(r)  "<r>"
  Bus Creator/1 -> FA_W/q/1
  Gain5/1 -> Bus Creator/3  "CL"
  Subsystem1/1("CY ") -> Bus Creator/2  "CY"
  Gain4/1 -> Bus Creator/1  "CD"

== system v2021_10_27_modello_calcolo_trim_1_semplificato/AENEA II /Forze aerodinamiche1/Momenti //press din ==
  Vect_Comandi : Inport
  Vect_Costanti : Inport  Port=2
  "Vbpolare " : Inport  Port=3
  ωb : Inport  Port=4
  Bus Creator : BusCreator  Inputs=3
  Bus Selector : BusSelector  OutputSignals=Coef_Geometrici.S*b,Coef_Geometrici.S*cbar
  Product : Product
  Product1 : Product
  Product3 : Product
  Subsystem3 : Subsystem
  Subsystem4 : Subsystem
  Subsystem5 : Subsystem
  MA_B/q : Outport  VectorParamsAs1DForOutWhenUnconnected=off
  wires:
  Subsystem5/1(Cn) -> Product3/2
  Subsystem4/1(Cm) -> Product1/2
  Subsystem3/1(Cl) -> Product/2
  Vect_Costanti/1 -> Bus Selector/1, Subsystem3/1(Vect_Costanti), Subsystem5/1(Vect_Costanti), Subsystem4/1(Vect_Costanti)
  Vect_Comandi/1 -> Subsystem4/2(Vect_Comandi), Subsystem3/2(Vect_Comandi), Subsystem5/2(Vect_Comandi)
  "Vbpolare "/1 -> Subsystem5/3("Vbpolare "), Subsystem4/3("Vbpolare "), Subsystem3/3("Vbpolare ")
  ωb/1 -> Subsystem5/4(ωb), Subsystem4/4(ωb), Subsystem3/4(ωb)
  Bus Selector/1 -> Product3/1, Product/1  "<S*b>"
  Bus Selector/2 -> Product1/1  "<S*cbar>"
  Bus Creator/1 -> MA_B/q/1
  Product/1 -> Bus Creator/1  "Cl"
  Product1/1 -> Bus Creator/2  "Cm"
  Product3/1 -> Bus Creator/3  "Cn"

== system v2021_10_27_modello_calcolo_trim_1_semplificato/AENEA II /Propulsione1/LUT ELICA  ==
  J : Inport
  RPM : Inport  Port=2
  2-D Lookup Table : Lookup_n-D  BreakpointsForDimension1=J_vec  BreakpointsForDimension2=RPM_vec(2:end)  Table=Ct(2:end,2:end)  InternalRulePriority=Speed  RndMeth=Simplest  InputSameDT=on
      settings: InputPortMap=u0,u1
  2-D Lookup Table1 : Lookup_n-D  BreakpointsForDimension1=J_vec  BreakpointsForDimension2=RPM_vec(2:end)  Table=Cp(2:end,2:end)  InternalRulePriority=Speed  RndMeth=Simplest  InputSameDT=on
      settings: InputPortMap=u0,u1
  Ct : Outport  VectorParamsAs1DForOutWhenUnconnected=off
  Cp : Outport  Port=2  VectorParamsAs1DForOutWhenUnconnected=off
  wires:
  RPM/1 -> 2-D Lookup Table/2, 2-D Lookup Table1/2
  J/1 -> 2-D Lookup Table1/1, 2-D Lookup Table/1
  2-D Lookup Table1/1 -> Cp/1
  2-D Lookup Table/1 -> Ct/1

== system v2021_10_27_modello_calcolo_trim_1_semplificato/AENEA II /Propulsione1/LUT ELICA 1 ==
  J : Inport
  RPM : Inport  Port=2
  Constant : Constant  Value=matricepolinomi  VectorParams1D=off
  MATLAB Function : MATLAB Function  TreatAsAtomicUnit=on
  Ct : Outport  VectorParamsAs1DForOutWhenUnconnected=off
  Cp : Outport  Port=2  VectorParamsAs1DForOutWhenUnconnected=off
  wires:
  MATLAB Function/2(Cp) -> Cp/1  "Cp"
  J/1 -> MATLAB Function/1(J)
  Constant/1 -> MATLAB Function/3(matricepolinomi)
  MATLAB Function/1(Ct) -> Ct/1  "Ct"
  RPM/1 -> MATLAB Function/2(RPM)

== system v2021_10_27_modello_calcolo_trim_1_semplificato/AENEA II /Propulsione1/Subsystem1 ==
  T : Inport
  P : Inport  Port=2
  RPS : Inport  Port=3
  V_cost : Inport  Port=4
  Bus Selector : BusSelector  OutputSignals=Coef_Propulsivi.Zeng
  Constant : Constant  Value=0
  Constant1 : Constant  Value=0
  Divide : Product  Inputs=*/
  Divide1 : Product  Inputs=**
  Gain : Gain  Gain=2*pi
  Gain1 : Gain  Gain=-1
  Mux : Mux  Inputs=3
  Mux1 : Mux  Inputs=3
  Fthrust : Outport  VectorParamsAs1DForOutWhenUnconnected=off
  "Mthrust " : Outport  Port=2  VectorParamsAs1DForOutWhenUnconnected=off
  wires:
  T/1 -> Divide1/2, Mux/1
  Constant/1 -> Mux/2, Mux/3
  Mux/1 -> Fthrust/1
  RPS/1 -> Gain/1
  P/1 -> Divide/1
  Gain/1 -> Divide/2
  Gain1/1 -> Mux1/1
  Divide/1 -> Gain1/1
  Divide1/1 -> Mux1/2
  Constant1/1 -> Mux1/3
  Mux1/1 -> "Mthrust "/1
  V_cost/1 -> Bus Selector/1
  Bus Selector/1 -> Divide1/1  "<Zeng>"

== system v2021_10_27_modello_calcolo_trim_1_semplificato/AENEA II /Forze aerodinamiche/Forze assi vento//q/Subsystem ==
  note: CD=CD(alpha_x,beta)
  Vect_Costanti : Inport
  "Vbpolare " : Inport  Port=2
  2-D Lookup Table : Lookup_n-D  BreakpointsForDimension1=alphavec_rad  BreakpointsForDimension2=betavec_rad  Table=CD(2:end,2:end)  InternalRulePriority=Speed  RndMeth=Simplest  InputSameDT=on
      settings: InputPortMap=u0,u1
  Bus Selector : BusSelector  OutputSignals=Coef_Aerodinamici.Coef_Forze.CD0
  Bus Selector1 : BusSelector  OutputSignals=α,β
  Sum1 : Sum  Inputs=|++
  CD : Outport  VectorParamsAs1DForOutWhenUnconnected=off
  wires:
  2-D Lookup Table/1 -> Sum1/1
  Sum1/1 -> CD/1
  Bus Selector/1 -> Sum1/2  "<CD0>"
  Vect_Costanti/1 -> Bus Selector/1
  Bus Selector1/1 -> 2-D Lookup Table/1  "<α>"
  "Vbpolare "/1 -> Bus Selector1/1
  Bus Selector1/2 -> 2-D Lookup Table/2  "<β>"

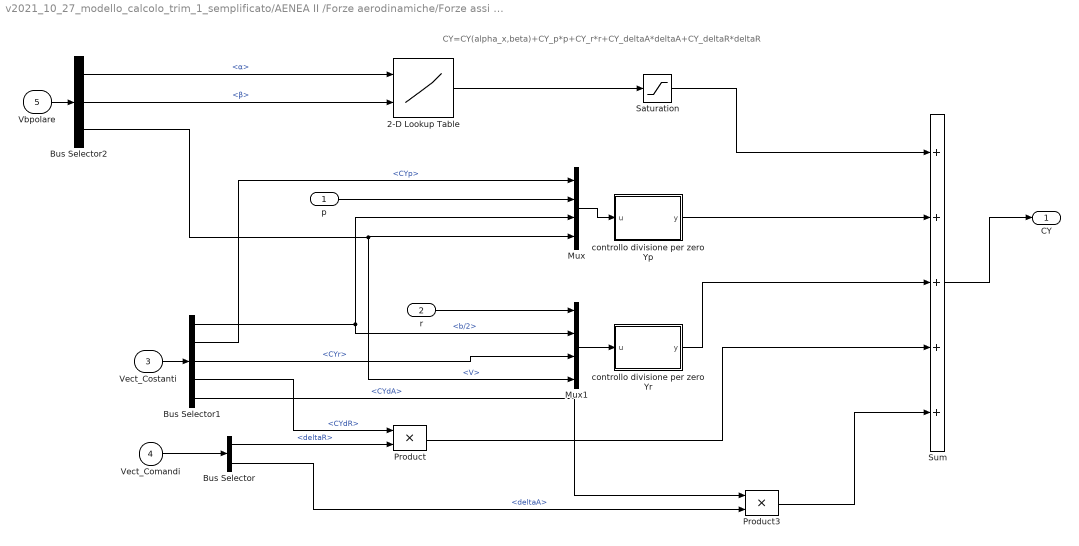
== system v2021_10_27_modello_calcolo_trim_1_semplificato/AENEA II /Forze aerodinamiche/Forze assi vento//q/Subsystem1 ==
  note: CY=CY(alpha_x,beta)+CY_p*p+CY_r*r+CY_deltaA*deltaA+CY_deltaR*deltaR
  p : Inport
  r : Inport  Port=2
  Vect_Costanti : Inport  Port=3
  Vect_Comandi : Inport  Port=4
  "Vbpolare " : Inport  Port=5
  2-D Lookup Table : Lookup_n-D  BreakpointsForDimension1=alphavec_rad  BreakpointsForDimension2=betavec_rad  Table=CY(2:end,2:end)  InternalRulePriority=Speed  RndMeth=Simplest  InputSameDT=on
      settings: InputPortMap=u0,u1
  Bus Selector : BusSelector  OutputSignals=deltaR,deltaA
  Bus Selector1 : BusSelector  OutputSignals=Coef_Geometrici.b/2,Coef_Aerodinamici.Coef_Forze.CYp,Coef_Aerodinamici.Coef_Forze.CYr,Coef_Aerodinamici.Coef_Forze.CYdR,Coef_Aerodinamici.Coef_Forze.CYdA
  Bus Selector2 : BusSelector  OutputSignals=α,β,V
  Mux : Mux
  Mux1 : Mux
  Product : Product
  Product3 : Product
  Saturation : Saturate  UpperLimit=0.1  LowerLimit=-0.1
  Sum : Sum  Inputs=5
  "controllo divisione per zero Yp " : MATLAB Function  TreatAsAtomicUnit=on
  controllo divisione per zero Yr : MATLAB Function  TreatAsAtomicUnit=on
  "CY " : Outport  VectorParamsAs1DForOutWhenUnconnected=off
  wires:
  Bus Selector1/2 -> Mux/1  "<CYp>"
  p/1 -> Mux/2
  "controllo divisione per zero Yp "/1(y) -> Sum/2
  Sum/1 -> "CY "/1
  r/1 -> Mux1/1
  2-D Lookup Table/1 -> Saturation/1
  Bus Selector1/4 -> Product/1  "<CYdR>"
  Bus Selector/1 -> Product/2  "<deltaR>"
  Bus Selector1/5 -> Product3/1  "<CYdA>"
  Bus Selector/2 -> Product3/2  "<deltaA>"
  Product/1 -> Sum/4
  Product3/1 -> Sum/5
  Vect_Comandi/1 -> Bus Selector/1
  Vect_Costanti/1 -> Bus Selector1/1
  Bus Selector1/3 -> Mux1/3  "<CYr>"
  Bus Selector1/1 -> Mux/3, Mux1/2  "<b/2>"
  Bus Selector2/1 -> 2-D Lookup Table/1  "<α>"
  "Vbpolare "/1 -> Bus Selector2/1
  Bus Selector2/3 -> Mux/4, Mux1/4  "<V>"
  Bus Selector2/2 -> 2-D Lookup Table/2  "<β>"
  Mux/1 -> "controllo divisione per zero Yp "/1(u)
  Mux1/1 -> controllo divisione per zero Yr/1(u)
  controllo divisione per zero Yr/1(y) -> Sum/3
  Saturation/1 -> Sum/1

== system v2021_10_27_modello_calcolo_trim_1_semplificato/AENEA II /Forze aerodinamiche/Forze assi vento//q/Subsystem2 ==
  note: CL=CL(ALPHA_X,BETA)+CL_q*q+CL_de*de
  q : Inport
  deltaE : Inport  Port=2
  Vect_Costanti : Inport  Port=3
  "Vbpolare " : Inport  Port=4
  2-D Lookup Table : Lookup_n-D  BreakpointsForDimension1=alphavec_rad  BreakpointsForDimension2=betavec_rad  Table=CL(2:end,2:end)  InternalRulePriority=Speed  RndMeth=Simplest  InputSameDT=on
      settings: InputPortMap=u0,u1
  Bus Selector : BusSelector  OutputSignals=Coef_Aerodinamici.Coef_Forze.CLq,Coef_Aerodinamici.Coef_Forze.CLdE,Coef_Geometrici.cbar
  Bus Selector1 : BusSelector  OutputSignals=α,β,V
  Gain1 : Gain  Gain=2
  Mux : Mux
  Product4 : Product
  Sum : Sum  Inputs=3
  "controllo divisione per zero Lq " : MATLAB Function  TreatAsAtomicUnit=on
  CL : Outport  VectorParamsAs1DForOutWhenUnconnected=off
  wires:
  Sum/1 -> CL/1
  q/1 -> Mux/2
  Bus Selector/1 -> Mux/1  "<CLq>"
  Bus Selector/2 -> Product4/1  "<CLdE>"
  deltaE/1 -> Product4/2
  "controllo divisione per zero Lq "/1(y) -> Sum/2
  Product4/1 -> Sum/3
  2-D Lookup Table/1 -> Sum/1
  Vect_Costanti/1 -> Bus Selector/1
  Gain1/1 -> Mux/4
  Bus Selector/3 -> Mux/3  "<cbar>"
  Bus Selector1/1 -> 2-D Lookup Table/1  "<α>"
  "Vbpolare "/1 -> Bus Selector1/1
  Bus Selector1/3 -> Gain1/1  "<V>"
  Bus Selector1/2 -> 2-D Lookup Table/2  "<β>"
  Mux/1 -> "controllo divisione per zero Lq "/1(u)

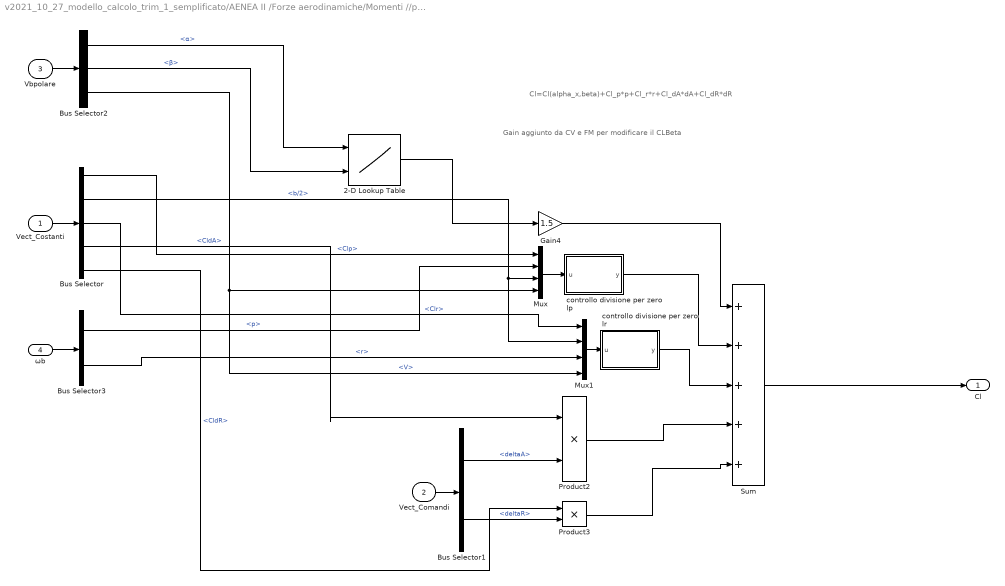
== system v2021_10_27_modello_calcolo_trim_1_semplificato/AENEA II /Forze aerodinamiche/Momenti //press din/Subsystem3 ==
  note: Gain aggiunto da CV e FM per modificare il CLBeta
  note: Cl=Cl(alpha_x,beta)+Cl_p*p+Cl_r*r+Cl_dA*dA+Cl_dR*dR
  Vect_Costanti : Inport
  Vect_Comandi : Inport  Port=2
  "Vbpolare " : Inport  Port=3
  ωb : Inport  Port=4
  2-D Lookup Table : Lookup_n-D  BreakpointsForDimension1=alphavec_rad  BreakpointsForDimension2=betavec_rad  Table=Cl(2:end,2:end)  InternalRulePriority=Speed  RndMeth=Simplest  InputSameDT=on
      settings: InputPortMap=u0,u1
  Bus Selector : BusSelector  OutputSignals=Coef_Aerodinamici.Coef_Momenti.Clp,Coef_Geometrici.b/2,Coef_Aerodinamici.Coef_Momenti.Clr,Coef_Aerodinamici.Coef_Momenti.CldA,Coef_Aerodinamici.Coef_Momenti.CldR
  Bus Selector1 : BusSelector  OutputSignals=deltaA,deltaR
  Bus Selector2 : BusSelector  OutputSignals=α,β,V
  Bus Selector3 : BusSelector  OutputSignals=p,r
  Gain4 : Gain  Gain=1.5
  Mux : Mux
  Mux1 : Mux
  Product2 : Product
  Product3 : Product
  Sum : Sum  Inputs=5
  "controllo divisione per zero lp " : MATLAB Function  TreatAsAtomicUnit=on
  "controllo divisione per zero lr " : MATLAB Function  TreatAsAtomicUnit=on
  Cl : Outport  VectorParamsAs1DForOutWhenUnconnected=off
  wires:
  Sum/1 -> Cl/1
  Bus Selector/3 -> Mux1/1  "<Clr>"
  Bus Selector1/2 -> Product3/2  "<deltaR>"
  Bus Selector1/1 -> Product2/2  "<deltaA>"
  Product3/1 -> Sum/5
  Product2/1 -> Sum/4
  "controllo divisione per zero lp "/1(y) -> Sum/2
  2-D Lookup Table/1 -> Gain4/1
  Gain4/1 -> Sum/1
  Vect_Costanti/1 -> Bus Selector/1
  Bus Selector/1 -> Mux/1  "<Clp>"
  Bus Selector/5 -> Product3/1  "<CldR>"
  Bus Selector/4 -> Product2/1  "<CldA>"
  Bus Selector/2 -> Mux1/2, Mux/3  "<b/2>"
  Vect_Comandi/1 -> Bus Selector1/1
  Bus Selector2/1 -> 2-D Lookup Table/1  "<α>"
  "Vbpolare "/1 -> Bus Selector2/1
  Bus Selector2/3 -> Mux1/4, Mux/4  "<V>"
  Bus Selector2/2 -> 2-D Lookup Table/2  "<β>"
  ωb/1 -> Bus Selector3/1
  Bus Selector3/1 -> Mux/2  "<p>"
  Bus Selector3/2 -> Mux1/3  "<r>"
  Mux/1 -> "controllo divisione per zero lp "/1(u)
  Mux1/1 -> "controllo divisione per zero lr "/1(u)
  "controllo divisione per zero lr "/1(y) -> Sum/3

== system v2021_10_27_modello_calcolo_trim_1_semplificato/AENEA II /Forze aerodinamiche/Momenti //press din/Subsystem4 ==
  note: Cm=Cm(alpha_x,beta)+Cmq*q+Cm_deltaE*deltaE
  Vect_Costanti : Inport
  Vect_Comandi : Inport  Port=2
  "Vbpolare " : Inport  Port=3
  ωb : Inport  Port=4
  2-D Lookup Table : Lookup_n-D  BreakpointsForDimension1=alphavec_rad  BreakpointsForDimension2=betavec_rad  Table=Cm(2:end,2:end)  InternalRulePriority=Speed  RndMeth=Simplest  InputSameDT=on
      settings: InputPortMap=u0,u1
  Bus Selector : BusSelector  OutputSignals=deltaE
  Bus Selector1 : BusSelector  OutputSignals=Coef_Geometrici.cbar,Coef_Aerodinamici.Coef_Momenti.Cmq,Coef_Aerodinamici.Coef_Momenti.CmdE
  Bus Selector2 : BusSelector  OutputSignals=α,β,V
  Bus Selector3 : BusSelector  OutputSignals=q
  Gain1 : Gain  Gain=2
  Mux : Mux
  Product2 : Product
  Sum : Sum  Inputs=3
  "controllo divisione per zero mq " : MATLAB Function  TreatAsAtomicUnit=on
  Cm : Outport  VectorParamsAs1DForOutWhenUnconnected=off
  wires:
  Bus Selector1/2 -> Mux/1  "<Cmq>"
  Sum/1 -> Cm/1
  Gain1/1 -> Mux/4
  Bus Selector1/3 -> Product2/1  "<CmdE>"
  Bus Selector/1 -> Product2/2  "<deltaE>"
  Product2/1 -> Sum/3
  2-D Lookup Table/1 -> Sum/1
  Vect_Comandi/1 -> Bus Selector/1
  Vect_Costanti/1 -> Bus Selector1/1
  Bus Selector1/1 -> Mux/3  "<cbar>"
  Bus Selector2/3 -> Gain1/1  "<V>"
  "Vbpolare "/1 -> Bus Selector2/1
  Bus Selector2/1 -> 2-D Lookup Table/1  "<α>"
  Bus Selector2/2 -> 2-D Lookup Table/2  "<β>"
  ωb/1 -> Bus Selector3/1
  Bus Selector3/1 -> Mux/2  "<q>"
  Mux/1 -> "controllo divisione per zero mq "/1(u)
  "controllo divisione per zero mq "/1(y) -> Sum/2

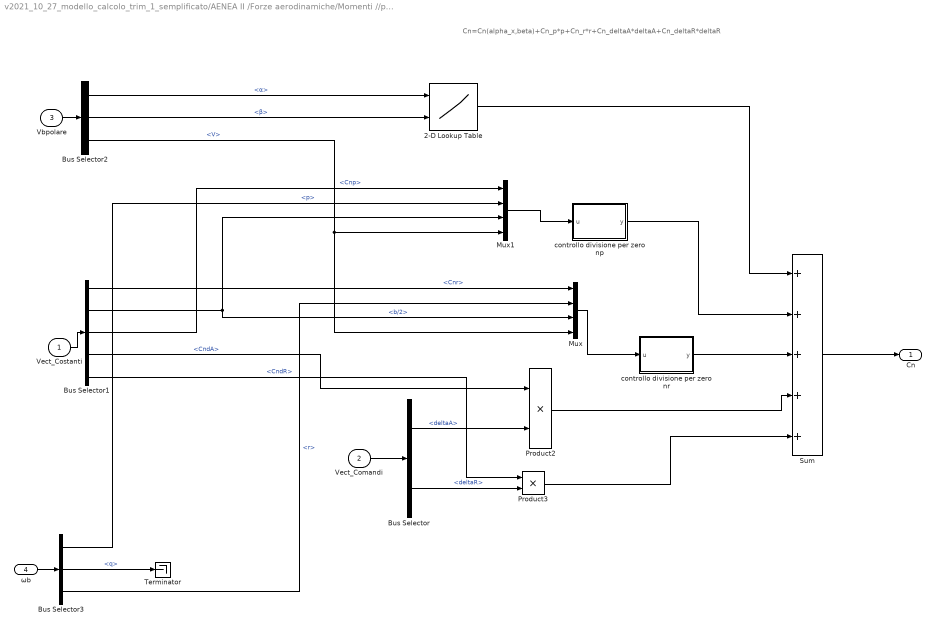
== system v2021_10_27_modello_calcolo_trim_1_semplificato/AENEA II /Forze aerodinamiche/Momenti //press din/Subsystem5 ==
  note: Cn=Cn(alpha_x,beta)+Cn_p*p+Cn_r*r+Cn_deltaA*deltaA+Cn_deltaR*deltaR
  Vect_Costanti : Inport
  Vect_Comandi : Inport  Port=2
  "Vbpolare " : Inport  Port=3
  ωb : Inport  Port=4
  2-D Lookup Table : Lookup_n-D  BreakpointsForDimension1=alphavec_rad  BreakpointsForDimension2=betavec_rad  Table=Cn(2:end,2:end)  InternalRulePriority=Speed  RndMeth=Simplest  InputSameDT=on
      settings: InputPortMap=u0,u1
  Bus Selector : BusSelector  OutputSignals=deltaA,deltaR
  Bus Selector1 : BusSelector  OutputSignals=Coef_Aerodinamici.Coef_Momenti.Cnr,Coef_Geometrici.b/2,Coef_Aerodinamici.Coef_Momenti.Cnp,Coef_Aerodinamici.Coef_Momenti.CndA,Coef_Aerodinamici.Coef_Momenti.CndR
  Bus Selector2 : BusSelector  OutputSignals=α,β,V
  Bus Selector3 : BusSelector  OutputSignals=p,q,r
  Mux : Mux
  Mux1 : Mux
  Product2 : Product
  Product3 : Product
  Sum : Sum  Inputs=5
  Terminator : Terminator
  "controllo divisione per zero np " : MATLAB Function  TreatAsAtomicUnit=on
  "controllo divisione per zero nr " : MATLAB Function  TreatAsAtomicUnit=on
  Cn : Outport  VectorParamsAs1DForOutWhenUnconnected=off
  wires:
  Bus Selector1/3 -> Mux1/1  "<Cnp>"
  Product2/1 -> Sum/4
  Product3/1 -> Sum/5
  Sum/1 -> Cn/1
  Bus Selector1/1 -> Mux/1  "<Cnr>"
  Bus Selector1/5 -> Product3/1  "<CndR>"
  Bus Selector/2 -> Product3/2  "<deltaR>"
  Bus Selector/1 -> Product2/2  "<deltaA>"
  2-D Lookup Table/1 -> Sum/1
  Vect_Comandi/1 -> Bus Selector/1
  Vect_Costanti/1 -> Bus Selector1/1
  Bus Selector1/4 -> Product2/1  "<CndA>"
  Bus Selector1/2 -> Mux1/3, Mux/3  "<b/2>"
  Bus Selector2/3 -> Mux1/4, Mux/4  "<V>"
  "Vbpolare "/1 -> Bus Selector2/1
  Bus Selector2/1 -> 2-D Lookup Table/1  "<α>"
  Bus Selector2/2 -> 2-D Lookup Table/2  "<β>"
  ωb/1 -> Bus Selector3/1
  Bus Selector3/3 -> Mux/2  "<r>"
  Bus Selector3/1 -> Mux1/2  "<p>"
  Bus Selector3/2 -> Terminator/1  "<q>"
  Mux/1 -> "controllo divisione per zero nr "/1(u)
  "controllo divisione per zero nr "/1(y) -> Sum/3
  Mux1/1 -> "controllo divisione per zero np "/1(u)
  "controllo divisione per zero np "/1(y) -> Sum/2

== system v2021_10_27_modello_calcolo_trim_1_semplificato/AENEA II /Forze aerodinamiche1/Forze assi vento//q/Subsystem ==
  note: CD=CD(alpha_x,beta)
  Vect_Costanti : Inport
  "Vbpolare " : Inport  Port=2
  2-D Lookup Table : Lookup_n-D  BreakpointsForDimension1=alphavec_rad  BreakpointsForDimension2=betavec_rad  Table=CD(2:end,2:end)  InternalRulePriority=Speed  RndMeth=Simplest  InputSameDT=on
      settings: InputPortMap=u0,u1
  Bus Selector : BusSelector  OutputSignals=Coef_Aerodinamici.Coef_Forze.CD0
  Bus Selector1 : BusSelector  OutputSignals=α,β
  Sum1 : Sum  Inputs=|++
  CD : Outport  VectorParamsAs1DForOutWhenUnconnected=off
  wires:
  2-D Lookup Table/1 -> Sum1/1
  Sum1/1 -> CD/1
  Bus Selector/1 -> Sum1/2  "<CD0>"
  Vect_Costanti/1 -> Bus Selector/1
  Bus Selector1/1 -> 2-D Lookup Table/1  "<α>"
  "Vbpolare "/1 -> Bus Selector1/1
  Bus Selector1/2 -> 2-D Lookup Table/2  "<β>"

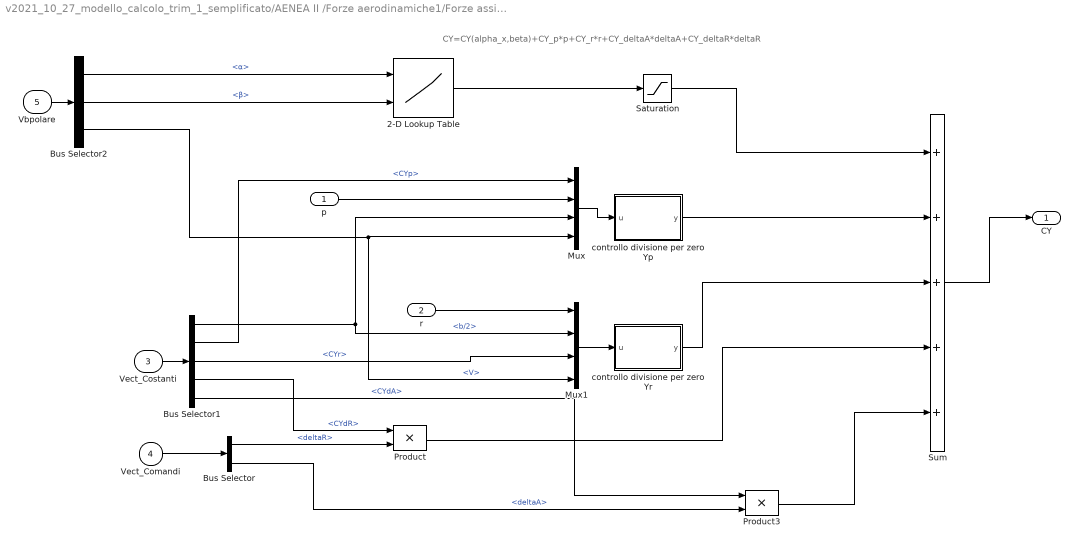
== system v2021_10_27_modello_calcolo_trim_1_semplificato/AENEA II /Forze aerodinamiche1/Forze assi vento//q/Subsystem1 ==
  note: CY=CY(alpha_x,beta)+CY_p*p+CY_r*r+CY_deltaA*deltaA+CY_deltaR*deltaR
  p : Inport
  r : Inport  Port=2
  Vect_Costanti : Inport  Port=3
  Vect_Comandi : Inport  Port=4
  "Vbpolare " : Inport  Port=5
  2-D Lookup Table : Lookup_n-D  BreakpointsForDimension1=alphavec_rad  BreakpointsForDimension2=betavec_rad  Table=CY(2:end,2:end)  InternalRulePriority=Speed  RndMeth=Simplest  InputSameDT=on
      settings: InputPortMap=u0,u1
  Bus Selector : BusSelector  OutputSignals=deltaR,deltaA
  Bus Selector1 : BusSelector  OutputSignals=Coef_Geometrici.b/2,Coef_Aerodinamici.Coef_Forze.CYp,Coef_Aerodinamici.Coef_Forze.CYr,Coef_Aerodinamici.Coef_Forze.CYdR,Coef_Aerodinamici.Coef_Forze.CYdA
  Bus Selector2 : BusSelector  OutputSignals=α,β,V
  Mux : Mux
  Mux1 : Mux
  Product : Product
  Product3 : Product
  Saturation : Saturate  UpperLimit=0.1  LowerLimit=-0.1
  Sum : Sum  Inputs=5
  "controllo divisione per zero Yp " : MATLAB Function  TreatAsAtomicUnit=on
  controllo divisione per zero Yr : MATLAB Function  TreatAsAtomicUnit=on
  "CY " : Outport  VectorParamsAs1DForOutWhenUnconnected=off
  wires:
  Bus Selector1/2 -> Mux/1  "<CYp>"
  p/1 -> Mux/2
  "controllo divisione per zero Yp "/1(y) -> Sum/2
  Sum/1 -> "CY "/1
  r/1 -> Mux1/1
  2-D Lookup Table/1 -> Saturation/1
  Bus Selector1/4 -> Product/1  "<CYdR>"
  Bus Selector/1 -> Product/2  "<deltaR>"
  Bus Selector1/5 -> Product3/1  "<CYdA>"
  Bus Selector/2 -> Product3/2  "<deltaA>"
  Product/1 -> Sum/4
  Product3/1 -> Sum/5
  Vect_Comandi/1 -> Bus Selector/1
  Vect_Costanti/1 -> Bus Selector1/1
  Bus Selector1/3 -> Mux1/3  "<CYr>"
  Bus Selector1/1 -> Mux/3, Mux1/2  "<b/2>"
  Bus Selector2/1 -> 2-D Lookup Table/1  "<α>"
  "Vbpolare "/1 -> Bus Selector2/1
  Bus Selector2/3 -> Mux/4, Mux1/4  "<V>"
  Bus Selector2/2 -> 2-D Lookup Table/2  "<β>"
  Mux/1 -> "controllo divisione per zero Yp "/1(u)
  Mux1/1 -> controllo divisione per zero Yr/1(u)
  controllo divisione per zero Yr/1(y) -> Sum/3
  Saturation/1 -> Sum/1
